simulink model "IonSatSimulationOld"  (R2019b)
settings: Solver=VariableStepAuto  StartTime=0.0  StopTime=10.0  RelTol=1e-3
model workspace (MAT data in the model file):
  Inertia = 1
undefined symbols (not defined in the file): I, mass
libraries: vrlib x1, qlib x1
settings Model: Creator=robin  LastModifiedBy=robin

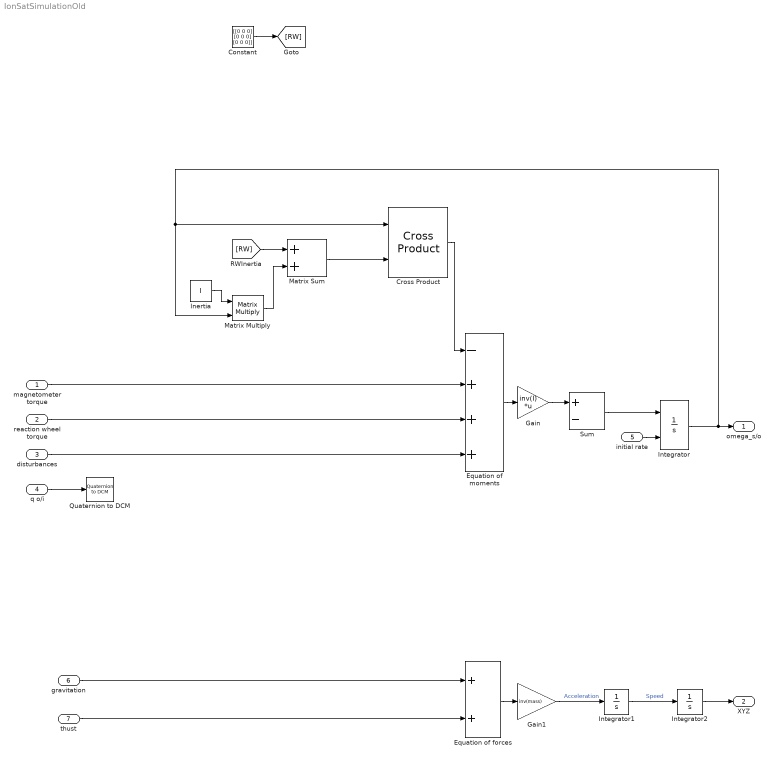
== system IonSatSimulationOld ==
  magnetometer torque : Inport
  reaction wheel torque : Inport  Port=2
  disturbances : Inport  Port=3
  q o/i : Inport  Port=4
  initial rate : Inport  Port=5
  gravitation : Inport  Port=6
  thust : Inport  Port=7
  Constant : Constant  Value=[[0 0 0] [0 0 0] [0 0 0]]  VectorParams1D=off
  Cross Product : vrlib/Utilities/Cross Product
      settings: SourceProductName=Simulink
  Equation of forces : Sum
  Equation of moments : Sum  Inputs=-+++
  Gain : Gain  Gain=inv(I)  Multiplication=Matrix(K*u)
  Gain1 : Gain  Gain=inv(mass)
  Inertia : Constant  Value=I
  Integrator : Integrator  InitialConditionSource=external
  Integrator1 : Integrator
  Integrator2 : Integrator
  Matrix Multiply : Product  Multiplication=Matrix(*)
  Matrix Sum : Sum
  Quaternion to DCM : qlib/Quaternion to DCM
  Sum : Sum  Inputs=+-
  omega_s/o : Outport
  XYZ : Outport  Port=2
  wires:
  gravitation/1 -> Equation of forces/1
  magnetometer torque/1 -> Equation of moments/2
  reaction wheel torque/1 -> Equation of moments/3
  disturbances/1 -> Equation of moments/4
  [RW] -> Matrix Sum/1
  Matrix Multiply/1 -> Matrix Sum/2
  Inertia/1 -> Matrix Multiply/1
  Integrator/1 -> Matrix Multiply/2, Cross Product/1, omega_s/o/1
  Equation of moments/1 -> Gain/1
  Matrix Sum/1 -> Cross Product/2
  Cross Product/1 -> Equation of moments/1
  Gain/1 -> Sum/1
  Sum/1 -> Integrator/1
  initial rate/1 -> Integrator/2
  Equation of forces/1 -> Gain1/1
  Gain1/1 -> Integrator1/1  "Acceleration"
  Integrator1/1 -> Integrator2/1  "Speed"
  Integrator2/1 -> XYZ/1
  thust/1 -> Equation of forces/2
  q o/i/1 -> Quaternion to DCM/1
  Constant/1 -> [RW]
